simulink model "sim_ex_1"  (Simulink 7.7)
settings: Solver=ode45  StartTime=0.0  StopTime=10.0  RelTol=1e-3
undefined symbols (not defined in the file or in its folder): degConv
settings Model: Creator=cjz  LastModifiedBy=cjz
settings DataIOCC: LoadExternalInput=on

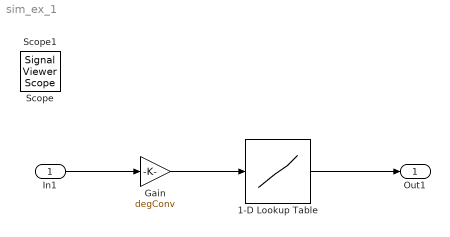
== system sim_ex_1 ==
  In1 : Inport
  1-D Lookup Table : Lookup_n-D  NumberOfTableDimensions=1  BreakpointsForDimension1=[0 90]  Table=[0.5 4.5]  RndMeth=Simplest  InputSameDT=on
  Gain : Gain  Gain=degConv
  Out1 : Outport
  Scope : SignalViewerScope  IOType=viewer  RefreshTime=0.035000
      settings: TimeRange=10  YMin=0  YMax=6
  Scope1 : SignalViewerScope  IOType=viewer  RefreshTime=0.035000
      settings: TimeRange=10  YMin=0  YMax=100
  wires:
  In1/1 -> Gain/1
  Gain/1 -> 1-D Lookup Table/1
  1-D Lookup Table/1 -> Out1/1
